simulink model "pipline_system"  (R2022b)
settings: Solver=FixedStepAuto  StartTime=0.0  StopTime=t_sim_stop  FixedStep=Tsim  RelTol=1e-3
values from neighbouring files (symbols this model uses):
  A_inv = pinv(Ad-eye(n),0.01)    [run_pipeline_system.m]    (also in run_pipeline_system_tree.m)
  Aeq = [A_bar -B_bar ... (first row only)    [run_pipeline_system.m]    (also in run_pipeline_system_tree.m)
  attack_final_deviations = 0.0*ones(n_meas,1)    [run_pipeline_system.m]    (also in run_pipeline_system_tree.m)
  attack_full_times = attack_start_times + 100    [run_pipeline_system.m]    (also in run_pipeline_system_tree.m)
  attack_start_times = attack_start_injection*ones(n_meas,1)    [run_pipeline_system.m]    (also in run_pipeline_system_tree.m)
  B = -[1;0;0;0;0;0;0;0;0;0;0]    [myStateTransitionFcnTopology.m]    (also in run_pipeline_system.m; run_pipeline_system_tree.m)
  B_dem = -[0;0;0;0;0;0;0;0;0;0;1]    [myStateTransitionFcnTopology.m]    (also in run_pipeline_system.m; run_pipeline_system_tree.m)
  B_demd = B_dem*Ts    [run_pipeline_system.m]    (also in run_pipeline_system_tree.m)
  B_h = -[0 0;0 0;0 0;1 0;0 0;0 0;0 0;0 1;0 0;0 0;0 0]    [myStateTransitionFcnTopology.m]    (also in run_pipeline_system.m; run_pipeline_system_tree.m)
  B_hd = B_h*Ts    [run_pipeline_system.m]    (also in run_pipeline_system_tree.m)
  c = 330    [myStateTransitionFcnTopology.m]    (also in run_pipeline_system.m; run_pipeline_system_tree.m)
  h = 10    [run_pipeline_system.m]    (also in run_pipeline_system_tree.m)
  K_inv = (pi^2)/(64*c^2)*f*D_edge.^5./L_edge    [myStateTransitionFcnTopology.m]    (also in run_pipeline_system.m; run_pipeline_system_tree.m)
  M = blkdiag(Q_bar, R_bar)    [run_pipeline_system.m]    (also in run_pipeline_system_tree.m)
  n = 11    [run_pipeline_system.m]    (also in run_pipeline_system_tree.m)
  n_meas = 14    [run_pipeline_system.m]    (also in run_pipeline_system_tree.m)
  p_eq = load("P_eq.mat").P_eq    [run_pipeline_system.m]    (also in run_pipeline_system_tree.m = load("P_eq_tree.mat").P_eq)
  p_init = p_eq    [run_pipeline_system.m]    (also in run_pipeline_system_tree.m)
  Q = 1e-5    (= 1e-05)    [run_pipeline_system.m]    (also in run_pipeline_system_tree.m)
  R = 1e-5    (= 1e-05)    [run_pipeline_system.m]    (also in run_pipeline_system_tree.m)
  Tsim = 1e-3    (= 0.001)    [run_pipeline_system.m]    (also in run_pipeline_system_tree.m)
  V = (pi/8)*sum(((D_edge.^2).*L_edge),2,'omitnan')    [myStateTransitionFcnTopology.m]    (also in run_pipeline_system.m; run_pipeline_system_tree.m)
  w_eq = [-1; -5; -5; 20]    [run_pipeline_system.m]    (also in run_pipeline_system_tree.m)
libraries: simulink x4, sharedTrackingLibrary x1
settings Model: Creator=RASLab-Distributed  LastModifiedBy=satis

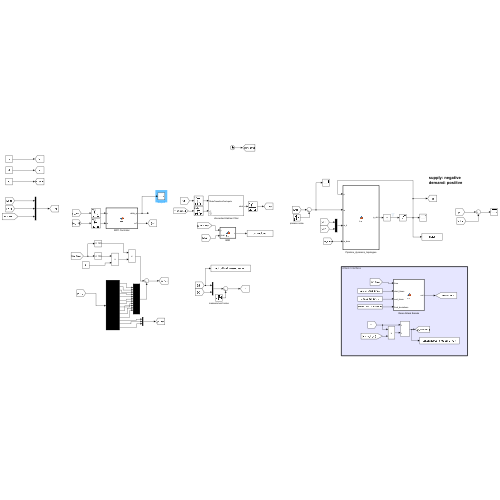
[thumbnail: Simulink's stored preview of the top-level diagram]
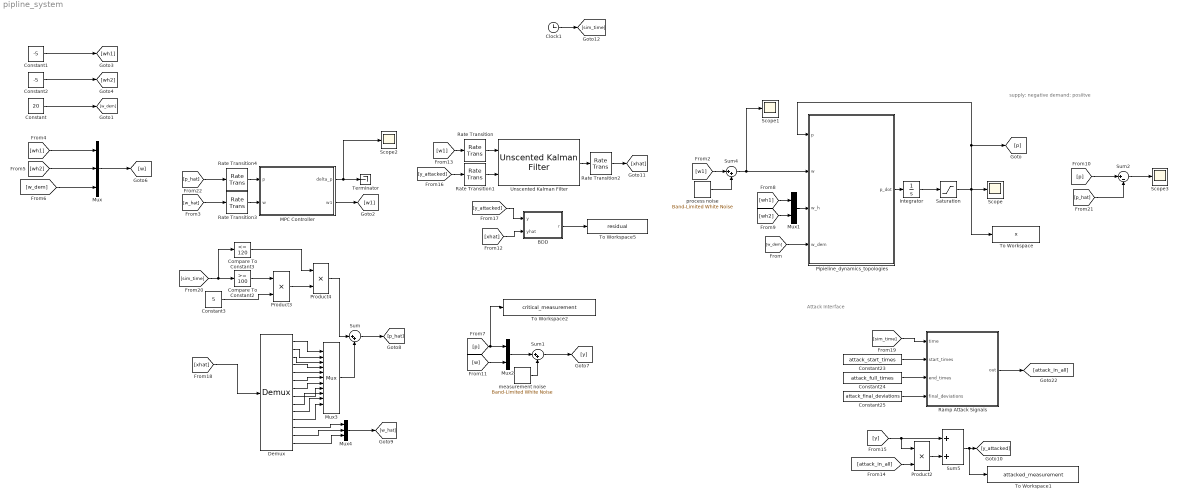
== system pipline_system ==
  note: supply: negative
      | demand: posiitve
  note: Attack Interface
  BDD : MATLAB Function  TreatAsAtomicUnit=on
  Clock1 : Clock
  Compare To Constant2 : simulink/Logic and Bit Operations/Compare To Constant  relop=>=  const=100  OutDataTypeStr=boolean
  Compare To Constant3 : simulink/Logic and Bit Operations/Compare To Constant  relop=<=  const=120  OutDataTypeStr=boolean
  Constant : Constant  Value=20
  Constant1 : Constant  Value=-5
  Constant2 : Constant  Value=-5
  Constant23 : Constant  Value=attack_start_times
  Constant24 : Constant  Value=attack_full_times
  Constant25 : Constant  Value=attack_final_deviations
  Constant3 : Constant  Value=5
  Demux : Demux  Outputs=n_meas
  Integrator : Integrator  InitialCondition=p_init
  MPC Controller : MATLAB Function  TreatAsAtomicUnit=on
  Mux : Mux  Inputs=3
  Mux1 : Mux  Inputs=2
  Mux2 : Mux  Inputs=2
  Mux3 : Mux  Inputs=n
  Mux4 : Mux  Inputs=3
  Pipieline_dynamics_topologies : MATLAB Function  TreatAsAtomicUnit=on
  Product2 : Product
  Product3 : Product
  Product4 : Product
  Ramp Attack Signals : MATLAB Function  TreatAsAtomicUnit=on
  Rate Transition : RateTransition  InitialCondition=w_eq(1)  OutPortSampleTime=Tsim
  Rate Transition1 : RateTransition  InitialCondition=[w_eq(2:end); p_eq]  OutPortSampleTime=Tsim
  Rate Transition2 : RateTransition  InitialCondition=[w_eq(2:end); p_eq]  OutPortSampleTime=0
  Rate Transition3 : RateTransition  OutPortSampleTime=T_MPC
  Rate Transition4 : RateTransition  OutPortSampleTime=T_MPC
  Saturation : Saturate  UpperLimit=inf  LowerLimit=0
  Scope{,1..3} (4 alike) : Scope
  Sum : Sum  Inputs=|++
  Sum1 : Sum  Inputs=|++
  Sum2 : Sum  Inputs=|+-
  Sum4 : Sum  Inputs=|++
  Sum5 : Sum
  Terminator : Terminator
  To Workspace : ToWorkspace  VariableName=x  SaveFormat=Timeseries  SampleTime=-1
  To Workspace1 : ToWorkspace  VariableName=attacked_measurement  SaveFormat=Timeseries  SampleTime=-1
  To Workspace2 : ToWorkspace  VariableName=critical_measurement  SaveFormat=Timeseries  SampleTime=-1
  To Workspace5 : ToWorkspace  VariableName=residual  SaveFormat=Timeseries  SampleTime=-1
  Unscented Kalman Filter : sharedTrackingLibrary/Unscented Kalman Filter  StateTransitionFcn=myStateTransitionFcnTopology  HasAdditiveProcessNoise=Additive  ProcessNoise=Q*eye(n_meas)  HasTimeVaryingProcessNoise=off  HasStateTransitionFcnExtraArgument=1  InitialState=[p_eq; w_eq(2:end)]  InitialStateCovariance=1  Alpha=1e-3  Beta=2  Kappa=0  MeasurementFcn1=myMeasurementFcn  HasMeasurementEnablePort1=off  HasAdditiveMeasurementNoise1=Additive  MeasurementNoise1=R*eye(n_meas)  HasTimeVaryingMeasurementNoise1=off  HasMeasurementFcnExtraArgument1=0  HasMeasurementWrapping1=off  MeasurementFcn2=myMeasurementFcn  HasMeasurementEnablePort2=off  HasAdditiveMeasurementNoise2=Additive  MeasurementNoise2=1  HasTimeVaryingMeasurementNoise2=off  HasMeasurementFcnExtraArgument2=0  HasMeasurementWrapping2=off  MeasurementFcn3=myMeasurementFcn  HasMeasurementEnablePort3=off  HasAdditiveMeasurementNoise3=Additive  MeasurementNoise3=1  HasTimeVaryingMeasurementNoise3=off  HasMeasurementFcnExtraArgument3=0  HasMeasurementWrapping3=off  MeasurementFcn4=myMeasurementFcn  HasMeasurementEnablePort4=off  HasAdditiveMeasurementNoise4=Additive  MeasurementNoise4=1  HasTimeVaryingMeasurementNoise4=off  HasMeasurementFcnExtraArgument4=0  HasMeasurementWrapping4=off  MeasurementFcn5=myMeasurementFcn  HasMeasurementEnablePort5=off  HasAdditiveMeasurementNoise5=Additive  MeasurementNoise5=1  HasTimeVaryingMeasurementNoise5=off  HasMeasurementFcnExtraArgument5=0  HasMeasurementWrapping5=off  EnableMultirate=off  StateTransitionFcnSampleTime=1  MeasurementFcn1SampleTime=1  MeasurementFcn2SampleTime=1  MeasurementFcn3SampleTime=1  MeasurementFcn4SampleTime=1  MeasurementFcn5SampleTime=1  UseCurrentEstimator=on  OutputStateCovariance=off  DataType=double  SampleTime=Tsim  NumberOfMeasurements=1
      settings: LibrarySourceBlock=cstblocks/State Estimation/Unscented Kalman Filter
  measurement noise : simulink/Sources/Band-Limited White Noise  Cov=R*Tsim  Ts=0.1  seed=[23341]
  process noise : simulink/Sources/Band-Limited White Noise  Cov=R*Tsim  Ts=0.1  seed=[23341]
  wires:
  Pipieline_dynamics_topologies/1(p_dot) -> Integrator/1
  Constant1/1 -> [wh1]
  Constant2/1 -> [wh2]
  Mux1/1 -> Pipieline_dynamics_topologies/3(w_h)
  [wh1] -> Mux1/1
  [wh2] -> Mux1/2
  Constant/1 -> [w_dem]
  [w_dem] -> Pipieline_dynamics_topologies/4(w_dem)
  Integrator/1 -> Saturation/1
  MPC Controller/1(delta_p) -> Scope2/1, Terminator/1
  MPC Controller/2(w1) -> [w1]
  Mux/1 -> [w]
  [wh1] -> Mux/1
  [wh2] -> Mux/2
  [w_dem] -> Mux/3
  [w_hat] -> Rate Transition3/1
  Rate Transition4/1 -> MPC Controller/1(p)
  Rate Transition3/1 -> MPC Controller/2(w)
  Saturation/1 -> To Workspace/1, [p], Pipieline_dynamics_topologies/1(p), Scope/1
  [p_hat] -> Rate Transition4/1
  [y] -> Product2/1, Sum5/1
  Constant24/1 -> Ramp Attack Signals/3(end_times)
  [attack_in_all] -> Product2/2
  Constant25/1 -> Ramp Attack Signals/4(final_deviations)
  Ramp Attack Signals/1(out) -> [attack_in_all]
  Constant23/1 -> Ramp Attack Signals/2(start_times)
  [sim_time] -> Ramp Attack Signals/1(time)
  Sum5/1 -> To Workspace1/1, [y_attacked]
  Product2/1 -> Sum5/2
  Clock1/1 -> [sim_time]
  [w] -> Mux2/2
  measurement noise/1 -> Sum1/2
  Sum1/1 -> [y]
  Mux2/1 -> Sum1/1
  [w1] -> Rate Transition/1
  BDD/1(r) -> To Workspace5/1
  Rate Transition1/1 -> Unscented Kalman Filter/2
  [y_attacked] -> BDD/1(y)
  Unscented Kalman Filter/1 -> Rate Transition2/1
  Rate Transition2/1 -> [xhat]
  [xhat] -> BDD/2(yhat)
  Rate Transition/1 -> Unscented Kalman Filter/1
  [y_attacked] -> Rate Transition1/1
  Compare To Constant3/1 -> Product4/1
  Product4/1 -> Sum/1
  Mux4/1 -> [w_hat]
  Product3/1 -> Product4/2
  Mux3/1 -> Sum/2
  Compare To Constant2/1 -> Product3/1
  Constant3/1 -> Product3/2
  [xhat] -> Demux/1
  [sim_time] -> Compare To Constant3/1, Compare To Constant2/1
  Sum/1 -> [p_hat]
  [p] -> Sum2/1
  [p_hat] -> Sum2/2
  Sum2/1 -> Scope3/1
  Sum4/1 -> Scope1/1, Pipieline_dynamics_topologies/2(w)
  [p] -> To Workspace2/1, Mux2/1
  process noise/1 -> Sum4/2
  [w1] -> Sum4/1
  Demux/1 -> Mux3/1
  Demux/2 -> Mux3/2
  Demux/3 -> Mux3/3
  Demux/4 -> Mux3/4
  Demux/5 -> Mux3/5
  Demux/6 -> Mux3/6
  Demux/7 -> Mux3/7
  Demux/8 -> Mux3/8
  Demux/9 -> Mux3/9
  Demux/10 -> Mux3/10
  Demux/11 -> Mux3/11
  Demux/12 -> Mux4/1
  Demux/13 -> Mux4/2
  Demux/14 -> Mux4/3

== matlab function pipline_system/Pipieline_dynamics_topologies ==
  data: p input; p_dot output; w input; w_h input; w_dem input; K_inv parameter; c parameter; V parameter; B_h parameter; B_dem parameter; B parameter
function p_dot = fcn(p,w,w_h,w_dem,K_inv, c, V, B_h, B_dem, B)
% COMMENTS HERE

p_sq = p.^2;
l    = ones(length(p),1);  % vector of ones
Psi = sqrt(K_inv.*abs(l*p_sq.' - p_sq*l.')).*sign(l*p.' - p*l.');

p_dot = c^2*(Psi*l)./V + B_h*w_h + B_dem*w_dem + B*w;

== matlab function pipline_system/MPC Controller ==
  data: delta_p output; p input; w input; w1 output; p_eq parameter; w_eq parameter; M parameter; Aeq parameter; B_hd parameter; B_demd parameter; n parameter; h parameter; A_inv parameter
function [delta_p,w1] = fcn(p,w,p_eq, w_eq, M, Aeq, B_hd, B_demd, n, h,A_inv)

% coder.extrinsic('quad_prog_solver');

%% formulate rest MPC parameters
% feedforward term
delta_w = w-w_eq(2:4);
pw = A_inv*(B_hd*delta_w(1:2) + B_demd*delta_w(3));

% additional internal state
delta_p = p-p_eq + pw;

% equality constraint
% beq1 = [Bh_bar -B_dem_bar]*kron(ones(h,1),delta_w);
beq1 = zeros(n*h,1);
beq2 = delta_p;
beq3 = pw;
beq = [beq1; beq2; beq3];

% objective
F = [-M(1:n*(h+1),1:n*(h+1))*kron(ones(h+1,1),pw); zeros(h,1)];

%% call solver
z = zeros(size(M,1),1);   % z = [delta_p; delta_w]
% z(:) = quad_prog_solver(M,F,Aeq,beq);
N = [M Aeq.';
     Aeq zeros(size(Aeq,1))];

N_inv = pinv(N,0.01);
N_inv1 = N_inv(1:size(M,1),:);

z = N_inv1*[-F; beq];

delta_w1 = z(n*h+1);


%% add feedfowward term
w1 = delta_w1 + w_eq(1);

== matlab function pipline_system/Ramp Attack Signals ==
  data: time input; out output; start_times input; end_times input; final_deviations input
function out = fcn(time,start_times,end_times,final_deviations)

delta_times = max(end_times-start_times,0);
ramp_rates  = final_deviations./delta_times;

deviations = (time<=start_times).*zeros(size(delta_times)) ...
    + ((time>start_times) & (time<=end_times)).*(ramp_rates.*(time-start_times)) ...
    + (time>end_times).*(final_deviations);

out = deviations;

== matlab function pipline_system/BDD ==
  data: y input; r output; yhat input
function r = fcn(y,yhat)

r=norm(y-yhat,2);
